simulink model "capitol3pb4"  (R2013a)
settings: Solver=ode45  StartTime=0.0  StopTime=57600  RelTol=1e-3
undefined symbols (not defined in the file): des, gcbh
settings Model: Creator=user  LastModifiedBy=user

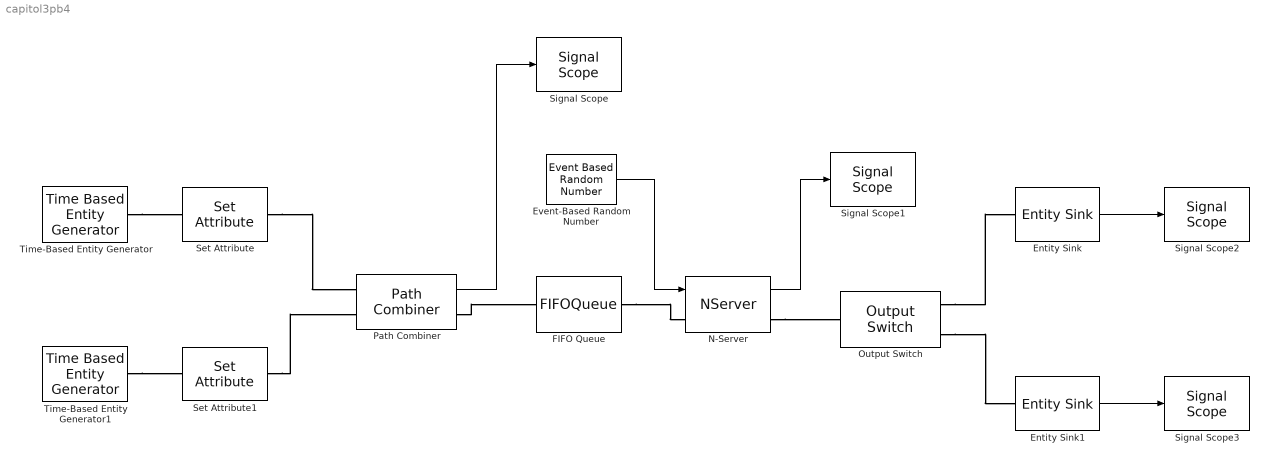
== system capitol3pb4 ==
  Entity Sink : EntitySink  StatNumberArrived=on
  Entity Sink1 : EntitySink  StatNumberArrived=on
  Event-Based Random Number : EventBasedRandomNumber  Distribution=Uniform  minUnif=840  maxUnif=1320
  FIFO Queue : FIFOQueue
  N-Server : NServer  NumberOfServers=2  ServiceTimeFrom=Signal port t  StatNumberDeparted=on
  Output Switch : OutputSwitch  NumberOutputPorts=2  SwitchingCriterion=From attribute
  Path Combiner : PathCombiner  NumberInputPorts=2  StatNumberDeparted=on
  Set Attribute : SetAttribute  EvaluatedAttributeValue={ 1}
  Set Attribute1 : SetAttribute  AttributeValue=2  EvaluatedAttributeValue={ 2}
  Signal Scope{,1..3} (4 alike) : SignalScope  LoadFcn=des.scope.CallbackSupport('seLoadFcn',gcbh)  StartFcn=des.scope.CallbackSupport('seStartFcn',gcbh)  StopFcn=des.scope.CallbackSupport('seStopFcn',gcbh)
      settings: CopyFcn=des.scope.CallbackSupport('seCopyFcn',gcbh)  DeleteFcn=des.scope.CallbackSupport('seDeleteFcn',gcbh)  PreSaveFcn=des.scope.CallbackSupport('sePreSaveFcn',gcbh)  NameChangeFcn=des.scope.CallbackSupport('seNameChangeFcn',gcbh)  OpenFcn=des.scope.CallbackSupport('seOpenFcn',gcbh)
  Time-Based Entity Generator : TimeBasedEntityGenerator  Distribution=Uniform  Minimum=1500  Maximum=2700  Mean=12
  Time-Based Entity Generator1 : TimeBasedEntityGenerator  Distribution=Uniform  Minimum=2280  Maximum=3120  Mean=12
  wires:
  Path Combiner/1 -> Signal Scope/1
  N-Server/1 -> Signal Scope1/1
  Event-Based Random Number/1 -> N-Server/1
  Entity Sink1/1 -> Signal Scope3/1
  Entity Sink/1 -> Signal Scope2/1
  connections:
  Time-Based Entity Generator/RConn1 -- Set Attribute/LConn1
  Time-Based Entity Generator1/RConn1 -- Set Attribute1/LConn1
  Set Attribute/RConn1 -- Path Combiner/LConn1
  Set Attribute1/RConn1 -- Path Combiner/LConn2
  Path Combiner/RConn1 -- FIFO Queue/LConn1
  FIFO Queue/RConn1 -- N-Server/LConn1
  N-Server/RConn1 -- Output Switch/LConn1
  Output Switch/RConn1 -- Entity Sink/LConn1
  Output Switch/RConn2 -- Entity Sink1/LConn1
